simulink model "ej2"  (R2020b)
settings: Solver=VariableStepAuto  StartTime=0.0  StopTime=10.0  RelTol=1e-3
settings Model: EnablePacing=on  Creator=Kike  LastModifiedBy=zunt7

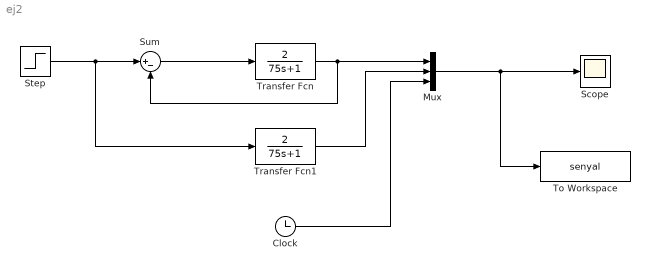
== system ej2 ==
  Clock : Clock
  Mux : Mux  Inputs=3
  Scope : Scope
  Step : Step  SampleTime=0
  Sum : Sum  Inputs=|+-
  To Workspace : ToWorkspace  VariableName=senyal  SaveFormat=Timeseries  SampleTime=-1
  Transfer Fcn : TransferFcn  Numerator=[2]  Denominator=[75 1]
  Transfer Fcn1 : TransferFcn  Numerator=[2]  Denominator=[75 1]
  wires:
  Step/1 -> Sum/1, Transfer Fcn1/1
  Sum/1 -> Transfer Fcn/1
  Transfer Fcn/1 -> Sum/2, Mux/1
  Transfer Fcn1/1 -> Mux/2
  Clock/1 -> Mux/3
  Mux/1 -> To Workspace/1, Scope/1
